simulink model "v2_3_debug5"  (R2017a)
settings: Solver=VariableStepAuto  StartTime=0.0  StopTime=50  RelTol=1e-3
values from neighbouring files (symbols this model uses):
  EbN0 = 18    [DataForResult.mat]
  TracebackDepth = 64    [DataForResult.mat]    (also in v2_3_1m.m; v2_3_debug0h.m; v2_3_debug1s.m; v2_3_debug2I.m)
libraries: commcnvcod2 x2, commblkintrlv2 x2, commchan3 x2, commdigbbndpm3 x1, commrandsrc3 x1, simulink x1, commsink2 x1
settings Model: Creator=DELL  LastModifiedBy=DELL

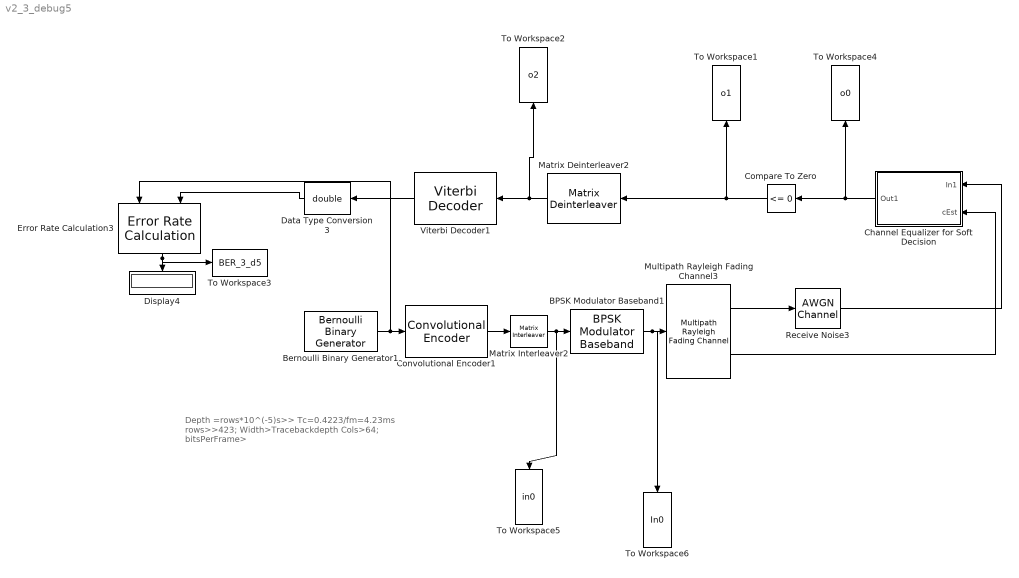
== system v2_3_debug5 ==
  note: Depth =rows*10^(-5)s>> Tc=0.4223/fm=4.23ms
      | 	rows>>423;
      |
      | Width>Tracebackdepth
      | 	Cols>64;
      |
      | bitsPerFrame>
  BPSK Modulator Baseband1 : commdigbbndpm3/BPSK Modulator Baseband  Ph=0  outDtype=double  outWordLen=16  outUDDataType=sfix(16)  outFracLenMode=Best precision  outFracLen=15  outDataTypeStr=double  outLastDataTypeStr=double
  Bernoulli Binary Generator1 : commrandsrc3/Bernoulli Binary Generator  ProbabilityOfZero=0.5  SeedSource=Auto  Seed=0  SampleTime=1e-5  SamplesPerFrame=SamplesPerFrame  OutputDataType=double  SimulateUsing=Interpreted execution
  Channel Equalizer for Soft Decision : Subsystem
      mask Display:
      | disp('Equalizer');
      | port_label('input', 2, 'cEst');
  Compare To Zero : simulink/Logic and Bit Operations/Compare To Zero  relop=<=  OutDataTypeStr=boolean
  Convolutional Encoder1 : commcnvcod2/Convolutional Encoder  trellis=poly2trellis(9, [561 753])  opMode=Continuous  DelayedResetAction=off  hasIniStPort=off  hasFinStPort=off  usePuncVector=off  punctureVector=[1; 1; 0; 1; 0; 1]  reset=Unused parameter value
      settings: SourceProductName=Communications System Toolbox  SourceProductBaseCode=CM
  Data Type Conversion3 : DataTypeConversion  OutDataTypeStr=double
  Display4 : Display
  Error Rate Calculation3 : commsink2/Error Rate Calculation  N=TracebackDepth  st_delay=0  cp_mode=Entire frame  subframe=[]  PMode=Port  WsName=ErrorVec  RsMode2=off  stop=off  numErr=100  maxBits=1e6
  Matrix Deinterleaver2 : commblkintrlv2/Matrix Deinterleaver  Nrows=Rows  Ncols=Cols
      settings: SourceProductName=Communications System Toolbox  SourceProductBaseCode=CM
  Matrix Interleaver2 : commblkintrlv2/Matrix Interleaver  Nrows=Rows  Ncols=Cols
      settings: SourceProductName=Communications System Toolbox  SourceProductBaseCode=CM
  Multipath Rayleigh Fading Channel3 : commchan3/Multipath Rayleigh Fading Channel  maxDopplerShift=100  spectrumType=Jakes  sigmaGaussian=1/sqrt(2)  coeffRounded=[1 -1.72 0.785]  freqMinMaxRJakes=[0 1]  freqMinMaxAJakes=[0 1]  sigmaGaussian1=1/sqrt(2)  sigmaGaussian2=1/sqrt(2)  centerFreqGaussian1=0.0  centerFreqGaussian2=0.0  gainGaussian1=0.5  gainGaussian2=0.5  coeffBell=9  dopplerSpectrum=doppler.jakes  pathDelays=0  avgPathGaindB=2  normalizePathGains=on  seed=12345  enableProbe=0  openVisAtStart=off  outPathGains=on  outDelay=off
      settings: SourceProductName=Communications System Toolbox  SourceProductBaseCode=CM
  Receive Noise3 : commchan3/AWGN Channel  InputProcessing=Columns as channels (frame based)  seed=188  noiseMode="Signal to noise ratio  (Eb/No)"  EbNodB=EbN0  EsNodB=EbNo  SNRdB=50  bitsPerSym=1  Ps=1  Tsym=1e-5  variance=1
  To Workspace1 : ToWorkspace  VariableName=o1  SampleTime=-1
      settings: MaxDataPoints=1
  To Workspace2 : ToWorkspace  VariableName=o2  SampleTime=-1
      settings: MaxDataPoints=1
  To Workspace3 : ToWorkspace  VariableName=BER_3_d5  SampleTime=-1
      settings: MaxDataPoints=1
  To Workspace4 : ToWorkspace  VariableName=o0  SampleTime=-1
      settings: MaxDataPoints=1
  To Workspace5 : ToWorkspace  VariableName=in0  SampleTime=-1
      settings: MaxDataPoints=1
  To Workspace6 : ToWorkspace  VariableName=In0  SampleTime=-1
      settings: MaxDataPoints=1
  Viterbi Decoder1 : commcnvcod2/Viterbi Decoder  trellis=poly2trellis(9, [561 753])  isPunctured=off  punctureVector=[1; 1; 0; 1; 0; 1]  erasures=off  dectype=Hard decision  nsdecb=1  runSigValErrCheck=off  tbdepth=TracebackDepth  opmode=Continuous  reset=off  delayedResetAction=off  smWordLength=16  outDataType=Inherit via internal rule
      settings: SourceProductName=Communications System Toolbox  SourceProductBaseCode=CM
  wires:
  BPSK Modulator Baseband1/1 -> To Workspace6/1, Multipath Rayleigh Fading Channel3/1
  Error Rate Calculation3/1 -> To Workspace3/1, Display4/1
  Multipath Rayleigh Fading Channel3/1 -> Receive Noise3/1
  Receive Noise3/1 -> Channel Equalizer for Soft Decision/1(In1)
  Data Type Conversion3/1 -> Error Rate Calculation3/2
  Bernoulli Binary Generator1/1 -> Error Rate Calculation3/1, Convolutional Encoder1/1
  Matrix Interleaver2/1 -> To Workspace5/1, BPSK Modulator Baseband1/1
  Matrix Deinterleaver2/1 -> To Workspace2/1, Viterbi Decoder1/1
  Convolutional Encoder1/1 -> Matrix Interleaver2/1
  Viterbi Decoder1/1 -> Data Type Conversion3/1
  Multipath Rayleigh Fading Channel3/2 -> Channel Equalizer for Soft Decision/2(cEst)
  Channel Equalizer for Soft Decision/1(Out1) -> To Workspace4/1, Compare To Zero/1
  Compare To Zero/1 -> To Workspace1/1, Matrix Deinterleaver2/1

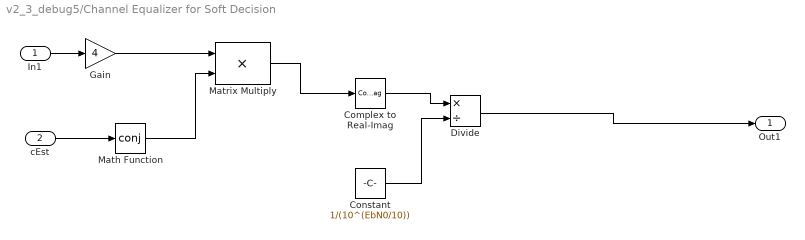
== system v2_3_debug5/Channel Equalizer for Soft Decision ==
  In1 : Inport
  cEst : Inport  Port=2
  Complex to Real-Imag : ComplexToRealImag  Output=Real
  Constant : Constant  Value=1/(10^(EbN0/10))
  Divide : Product  Inputs=*/
  Gain : Gain  Gain=4
  Math Function : Math  Operator=conj  SaturateOnIntegerOverflow=on
  Matrix Multiply : Product
  Out1 : Outport
  wires:
  In1/1 -> Gain/1
  cEst/1 -> Math Function/1
  Matrix Multiply/1 -> Complex to Real-Imag/1
  Math Function/1 -> Matrix Multiply/2
  Gain/1 -> Matrix Multiply/1
  Constant/1 -> Divide/2
  Complex to Real-Imag/1 -> Divide/1
  Divide/1 -> Out1/1
